simulink model "ISZM"  (R2025a)
settings: Solver=VariableStepAuto  StartTime=0.0  StopTime=1  MaxStep=1e-3  RelTol=1e-3
libraries: MSZSZ_MK x1
settings Model: Creator=Szalay  LastModifiedBy=Szalay

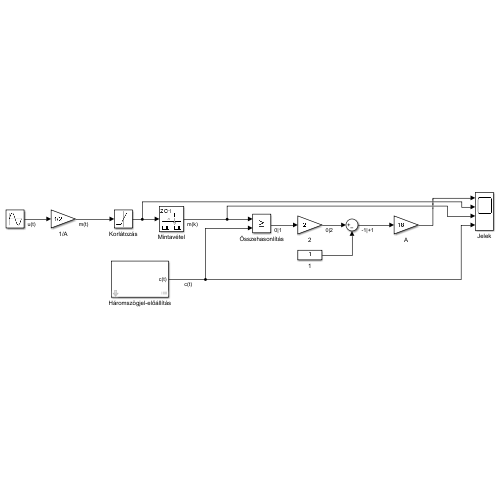
[thumbnail: Simulink's stored preview of the top-level diagram]
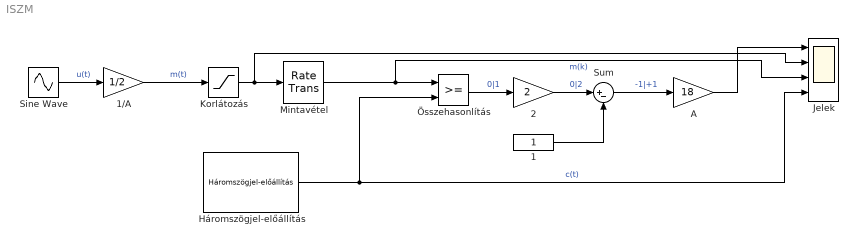
== system ISZM ==
  1 : Constant
  1/A : Gain  Gain=1/2
  2 : Gain  Gain=2
  A : Gain  Gain=18
  Háromszögjel-előállítás : MSZSZ_MK/Háromszögjel-előállítás  A=1  f=10  B=0
  Jelek : Scope  NumInputPorts=4
      settings: ActiveDisplayYMinimum=-22.5  ActiveDisplayYMaximum=22.5
  Korlátozás : Saturate  UpperLimit=0.95  LowerLimit=-0.95
  Mintavétel : RateTransition  OutPortSampleTime=1/10/2
  Sine Wave : Sin  Amplitude=2  Frequency=2*pi*1  SampleTime=0
  Sum : Sum  Inputs=|+-
  Összehasonlítás : RelationalOperator  OutDataTypeStr=boolean  RndMeth=Simplest  InputSameDT=off
  wires:
  Háromszögjel-előállítás/1 -> Jelek/4, Összehasonlítás/2  "c(t)"
  Mintavétel/1 -> Jelek/3, Összehasonlítás/1  "m(k)"
  Összehasonlítás/1 -> 2/1  "0|1"
  Sine Wave/1 -> 1/A/1  "u(t)"
  1/A/1 -> Korlátozás/1  "m(t)"
  Sum/1 -> A/1  "-1|+1"
  2/1 -> Sum/1  "0|2"
  1/1 -> Sum/2
  A/1 -> Jelek/1
  Korlátozás/1 -> Jelek/2, Mintavétel/1
